simulink model "ADRCControl_20220610"  (R2020a)
settings: Solver=VariableStepAuto  StartTime=0.0  StopTime=12  FixedStep=0.01  RelTol=1e-3
values from neighbouring files (symbols this model uses):
  alpha1 = 0.5    [parameters_initialization.m]
  alpha2 = 0.25    [parameters_initialization.m]
  b = 2    [parameters_initialization.m]
  beta01 = 6    [parameters_initialization.m]
  beta02 = 24    [parameters_initialization.m]
  beta03 = 4    [parameters_initialization.m]
  delta = 0.0025    [parameters_initialization.m]
  h = 0.01    [parameters_initialization.m]
  h0 = 5 * h    (= 0.05)    [parameters_initialization.m]
  nlsef_alpha1 = 0.7    [parameters_initialization.m]
  nlsef_alpha2 = 1    [parameters_initialization.m]
  r = 100    [parameters_initialization.m]
undefined symbols (not defined in the file or in its folder): X, Y, Z
libraries: sm_lib x197, nesl_utility x84, sm_cable_robot_lib x44, simulink x3
(part 1 of 9)
settings Model: Creator=admin  LastModifiedBy=Administrator
settings SolverCC: AlgebraicLoopSolver=LineSearch

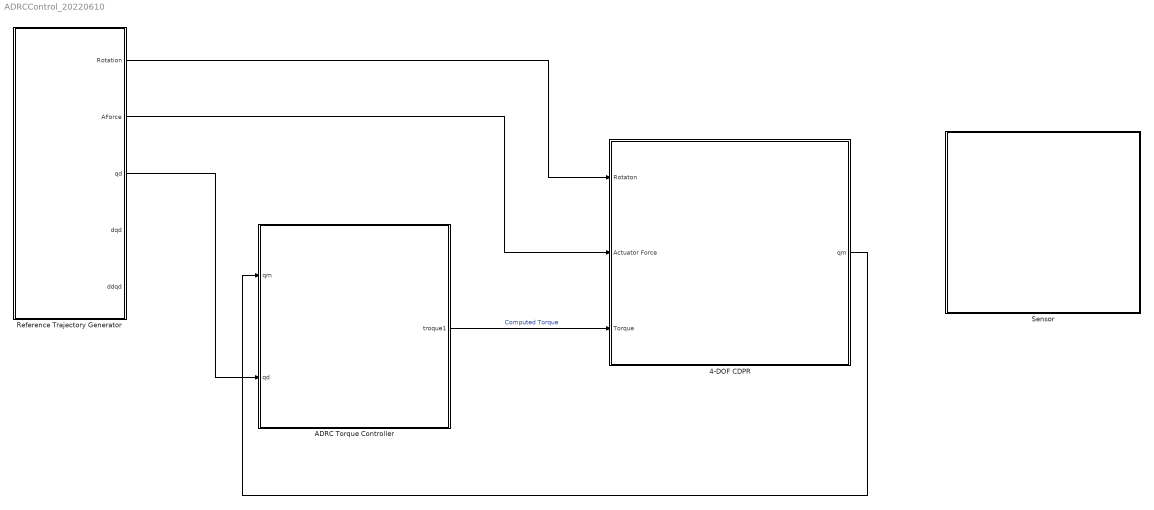
== system ADRCControl_20220610 ==
  4-DOF CDPR : Subsystem
  ADRC Torque Controller : Subsystem
  Reference Trajectory Generator : Subsystem
  Sensor : Subsystem
  wires:
  4-DOF CDPR/1(qm) -> ADRC Torque Controller/1(qm)
  Reference Trajectory Generator/1(Rotation) -> 4-DOF CDPR/1(Rotaton)
  Reference Trajectory Generator/2(AForce) -> 4-DOF CDPR/2("Actuator Force ")
  ADRC Torque Controller/1(troque1) -> 4-DOF CDPR/3(Torque)  "Computed Torque"
  Reference Trajectory Generator/3(qd) -> ADRC Torque Controller/2(qd)

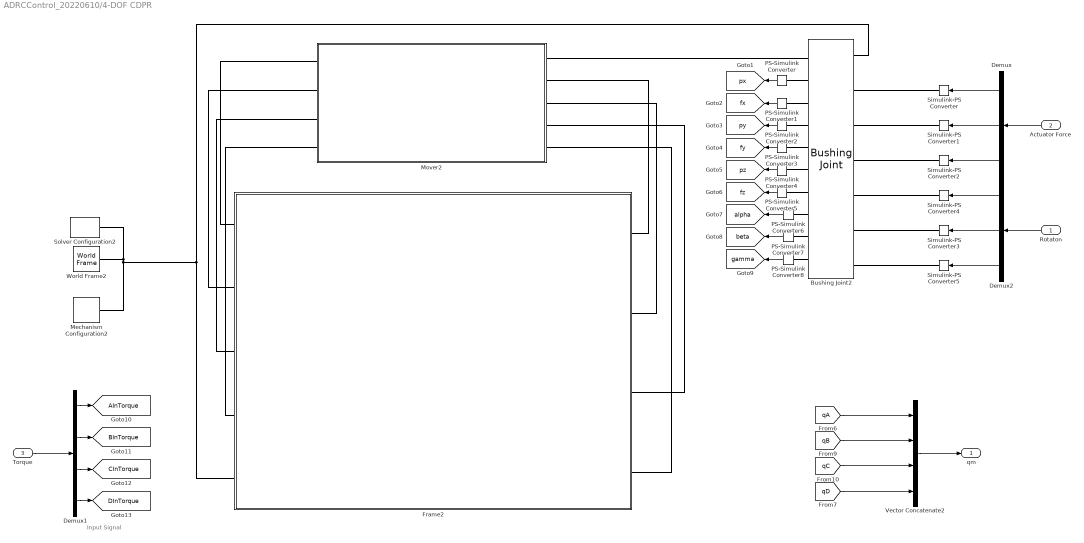
== system ADRCControl_20220610/4-DOF CDPR ==
  note: Input Signal
  Rotaton : Inport
  "Actuator Force " : Inport  Port=2
  Torque : Inport  Port=3
  Bushing Joint2 : sm_lib/Joints/Bushing Joint  JointMode=Normal  SenseConstraintForce=off  SenseConstraintForceX=off  SenseConstraintForceY=off  SenseConstraintForceZ=off  SenseConstraintTorque=off  SenseConstraintTorqueX=off  SenseConstraintTorqueY=off  SenseConstraintTorqueZ=off  SenseTotalForce=off  SenseTotalForceX=off  SenseTotalForceY=off  SenseTotalForceZ=off  SenseTotalTorque=off  SenseTotalTorqueX=off  SenseTotalTorqueY=off  SenseTotalTorqueZ=off  CompositeWrenchDir=FollowerOnBase  CompositeWrenchFrame=BaseFrame  PxEquilibriumPosition=0.2  PxEquilibriumPositionUnits=m  PxSpringStiffness=0  PxSpringStiffnessUnits=N/m  PxDampingCoefficient=0  PxDampingCoefficientUnits=N/(m/s)  PxTorqueActuationMode=InputTorque  PxMotionActuationMode=ComputedMotion  PxSensePosition=on  PxSenseVelocity=off  PxSenseAcceleration=off  PxSenseTorqueForce=on  PxSenseLowerLimitTorqueForce=off  PxSenseUpperLimitTorqueForce=off  PxLowerLimitSpecify=off  PxLowerLimitBound=-1  PxLowerLimitBoundUnits=m  PxLowerLimitStiffness=1e6  PxLowerLimitStiffnessUnits=N/m  PxLowerLimitDamping=1e3  PxLowerLimitDampingUnits=N/(m/s)  PxLowerLimitTransitionRegionWidth=1e-4  PxLowerLimitTransitionRegionWidthUnits=m  PxUpperLimitSpecify=off  PxUpperLimitBound=1  PxUpperLimitBoundUnits=m  PxUpperLimitStiffness=1e6  PxUpperLimitStiffnessUnits=N/m  PxUpperLimitDamping=1e3  PxUpperLimitDampingUnits=N/(m/s)  PxUpperLimitTransitionRegionWidth=1e-4  PxUpperLimitTransitionRegionWidthUnits=m  PxPositionTargetSpecify=on  PxPositionTargetPriority=Low  PxPositionTargetValue=0.2  PxPositionTargetValueUnits=m  PxVelocityTargetSpecify=off  PxVelocityTargetPriority=High  PxVelocityTargetValue=0.1047  PxVelocityTargetValueUnits=m/s  PyEquilibriumPosition=0  PyEquilibriumPositionUnits=m  PySpringStiffness=0  PySpringStiffnessUnits=N/m  PyDampingCoefficient=0  PyDampingCoefficientUnits=N/(m/s)  PyTorqueActuationMode=InputTorque  PyMotionActuationMode=ComputedMotion  PySensePosition=on  PySenseVelocity=off  PySenseAcceleration=off  PySenseTorqueForce=on  PySenseLowerLimitTorqueForce=off  PySenseUpperLimitTorqueForce=off  PyLowerLimitSpecify=off  PyLowerLimitBound=-1  PyLowerLimitBoundUnits=m  PyLowerLimitStiffness=1e6  PyLowerLimitStiffnessUnits=N/m  PyLowerLimitDamping=1e3  PyLowerLimitDampingUnits=N/(m/s)  PyLowerLimitTransitionRegionWidth=1e-4  PyLowerLimitTransitionRegionWidthUnits=m  PyUpperLimitSpecify=off  PyUpperLimitBound=1  PyUpperLimitBoundUnits=m  PyUpperLimitStiffness=1e6  PyUpperLimitStiffnessUnits=N/m  PyUpperLimitDamping=1e3  PyUpperLimitDampingUnits=N/(m/s)  PyUpperLimitTransitionRegionWidth=1e-4  PyUpperLimitTransitionRegionWidthUnits=m  PyPositionTargetSpecify=on  PyPositionTargetPriority=Low  PyPositionTargetValue=0  PyPositionTargetValueUnits=m  PyVelocityTargetSpecify=off  PyVelocityTargetPriority=High  PyVelocityTargetValue=0.1047  PyVelocityTargetValueUnits=m/s  PzEquilibriumPosition=1.3  PzEquilibriumPositionUnits=m  PzSpringStiffness=0  PzSpringStiffnessUnits=N/m  PzDampingCoefficient=0  PzDampingCoefficientUnits=N/(m/s)  PzTorqueActuationMode=InputTorque  PzMotionActuationMode=ComputedMotion  PzSensePosition=on  PzSenseVelocity=off  PzSenseAcceleration=off  PzSenseTorqueForce=on  PzSenseLowerLimitTorqueForce=off  PzSenseUpperLimitTorqueForce=off  PzLowerLimitSpecify=off  PzLowerLimitBound=-1  PzLowerLimitBoundUnits=m  PzLowerLimitStiffness=1e6  PzLowerLimitStiffnessUnits=N/m  PzLowerLimitDamping=1e3  PzLowerLimitDampingUnits=N/(m/s)  PzLowerLimitTransitionRegionWidth=1e-4  PzLowerLimitTransitionRegionWidthUnits=m  PzUpperLimitSpecify=off  PzUpperLimitBound=1  PzUpperLimitBoundUnits=m  PzUpperLimitStiffness=1e6  PzUpperLimitStiffnessUnits=N/m  PzUpperLimitDamping=1e3  PzUpperLimitDampingUnits=N/(m/s)  PzUpperLimitTransitionRegionWidth=1e-4  PzUpperLimitTransitionRegionWidthUnits=m  PzPositionTargetSpecify=on  PzPositionTargetPriority=Low  PzPositionTargetValue=1.3  PzPositionTargetValueUnits=m  PzVelocityTargetSpecify=off  PzVelocityTargetPriority=High  PzVelocityTargetValue=0  PzVelocityTargetValueUnits=m/s  RxEquilibriumPosition=0  RxEquilibriumPositionUnits=deg  RxSpringStiffness=0  RxSpringStiffnessUnits=N*m/deg  RxDampingCoefficient=0  RxDampingCoefficientUnits=N*m/(deg/s)  RxTorqueActuationMode=ComputedTorque  RxMotionActuationMode=InputMotion  RxSensePosition=on  RxSenseVelocity=off  RxSenseAcceleration=off  RxSenseTorqueForce=off  RxSenseLowerLimitTorqueForce=off  RxSenseUpperLimitTorqueForce=off  RxLowerLimitSpecify=off  RxLowerLimitBound=-90  RxLowerLimitBoundUnits=deg  RxLowerLimitStiffness=1e4  RxLowerLimitStiffnessUnits=N*m/deg  RxLowerLimitDamping=10  RxLowerLimitDampingUnits=N*m/(deg/s)  RxLowerLimitTransitionRegionWidth=0.1  RxLowerLimitTransitionRegionWidthUnits=deg  RxUpperLimitSpecify=off  RxUpperLimitBound=90  RxUpperLimitBoundUnits=deg  RxUpperLimitStiffness=1e4  RxUpperLimitStiffnessUnits=N*m/deg  RxUpperLimitDamping=10  RxUpperLimitDampingUnits=N*m/(deg/s)  RxUpperLimitTransitionRegionWidth=0.1  RxUpperLimitTransitionRegionWidthUnits=deg  RxPositionTargetSpecify=off  RxPositionTargetPriority=High  RxPositionTargetValue=0  RxPositionTargetValueUnits=deg  RxVelocityTargetSpecify=off  RxVelocityTargetPriority=High  RxVelocityTargetValue=0  RxVelocityTargetValueUnits=deg/s  RyEquilibriumPosition=0  RyEquilibriumPositionUnits=deg  RySpringStiffness=0  RySpringStiffnessUnits=N*m/deg  RyDampingCoefficient=0  RyDampingCoefficientUnits=N*m/(deg/s)  RyTorqueActuationMode=ComputedTorque  RyMotionActuationMode=InputMotion  RySensePosition=on  RySenseVelocity=off  RySenseAcceleration=off  RySenseTorqueForce=off  RySenseLowerLimitTorqueForce=off  RySenseUpperLimitTorqueForce=off  RyLowerLimitSpecify=off  RyLowerLimitBound=-90  RyLowerLimitBoundUnits=deg  RyLowerLimitStiffness=1e4  RyLowerLimitStiffnessUnits=N*m/deg  RyLowerLimitDamping=10  RyLowerLimitDampingUnits=N*m/(deg/s)  RyLowerLimitTransitionRegionWidth=0.1  RyLowerLimitTransitionRegionWidthUnits=deg  RyUpperLimitSpecify=off  RyUpperLimitBound=90  RyUpperLimitBoundUnits=deg  RyUpperLimitStiffness=1e4  RyUpperLimitStiffnessUnits=N*m/deg  RyUpperLimitDamping=10  RyUpperLimitDampingUnits=N*m/(deg/s)  RyUpperLimitTransitionRegionWidth=0.1  RyUpperLimitTransitionRegionWidthUnits=deg  RyPositionTargetSpecify=off  RyPositionTargetPriority=High  RyPositionTargetValue=0  RyPositionTargetValueUnits=deg  RyVelocityTargetSpecify=off  RyVelocityTargetPriority=High  RyVelocityTargetValue=0  RyVelocityTargetValueUnits=deg/s  RzEquilibriumPosition=0  RzEquilibriumPositionUnits=deg  RzSpringStiffness=0  RzSpringStiffnessUnits=N*m/deg  RzDampingCoefficient=0.01  RzDampingCoefficientUnits=N*m/(deg/s)  RzTorqueActuationMode=ComputedTorque  RzMotionActuationMode=InputMotion  RzSensePosition=on  RzSenseVelocity=off  RzSenseAcceleration=off  RzSenseTorqueForce=off  RzSenseLowerLimitTorqueForce=off  RzSenseUpperLimitTorqueForce=off  RzLowerLimitSpecify=off  RzLowerLimitBound=-90  RzLowerLimitBoundUnits=deg  RzLowerLimitStiffness=1e4  RzLowerLimitStiffnessUnits=N*m/deg  RzLowerLimitDamping=10  RzLowerLimitDampingUnits=N*m/(deg/s)  RzLowerLimitTransitionRegionWidth=0.1  RzLowerLimitTransitionRegionWidthUnits=deg  RzUpperLimitSpecify=off  RzUpperLimitBound=90  RzUpperLimitBoundUnits=deg  RzUpperLimitStiffness=1e4  RzUpperLimitStiffnessUnits=N*m/deg  RzUpperLimitDamping=10  RzUpperLimitDampingUnits=N*m/(deg/s)  RzUpperLimitTransitionRegionWidth=0.1  RzUpperLimitTransitionRegionWidthUnits=deg  RzPositionTargetSpecify=on  RzPositionTargetPriority=High  RzPositionTargetValue=0  RzPositionTargetValueUnits=deg  RzVelocityTargetSpecify=off  RzVelocityTargetPriority=High  RzVelocityTargetValue=0  RzVelocityTargetValueUnits=deg/s
  Demux : Demux  Outputs=3
  Demux1 : Demux
  Demux2 : Demux  Outputs=3
  Frame2 : Subsystem
  Mechanism Configuration2 : sm_lib/Utilities/Mechanism Configuration  UniformGravity=Constant  GravityVector=[0 0 -9.8]  GravityUnits=m/s^2  LinearizationDelta=0.001
  Mover2 : Subsystem
  PS-Simulink Converter{,1..8} (9 alike) : nesl_utility/PS-Simulink Converter  PhysicalDomain=network_engine_domain  SubClassName=ps_output  LeftPortType=input  RightPortType=output  PseudoPeriodic=off  Frequencies=[]  Unit=inherit  AffineConversion=off
  Simulink-PS Converter : nesl_utility/Simulink-PS Converter  PhysicalDomain=network_engine_domain  SubClassName=ps_input  LeftPortType=input  RightPortType=output  PseudoPeriodic=off  Frequencies=[]  NoiseDistribution=none  NoiseParameters=[]  Unit=N  AffineConversion=off  FilteringAndDerivatives=filter  SimscapeFilterOrder=2  InputFilterTimeConstant=0.001  UdotUserProvided=0
  Simulink-PS Converter1 : nesl_utility/Simulink-PS Converter  PhysicalDomain=network_engine_domain  SubClassName=ps_input  LeftPortType=input  RightPortType=output  PseudoPeriodic=off  Frequencies=[]  NoiseDistribution=none  NoiseParameters=[]  Unit=N  AffineConversion=off  FilteringAndDerivatives=filter  SimscapeFilterOrder=2  InputFilterTimeConstant=0.001  UdotUserProvided=0
  Simulink-PS Converter2 : nesl_utility/Simulink-PS Converter  PhysicalDomain=network_engine_domain  SubClassName=ps_input  LeftPortType=input  RightPortType=output  PseudoPeriodic=off  Frequencies=[]  NoiseDistribution=none  NoiseParameters=[]  Unit=N  AffineConversion=off  FilteringAndDerivatives=filter  SimscapeFilterOrder=2  InputFilterTimeConstant=0.001  UdotUserProvided=0
  Simulink-PS Converter3 : nesl_utility/Simulink-PS Converter  PhysicalDomain=network_engine_domain  SubClassName=ps_input  LeftPortType=input  RightPortType=output  PseudoPeriodic=off  Frequencies=[]  NoiseDistribution=none  NoiseParameters=[]  Unit=1  AffineConversion=off  FilteringAndDerivatives=filter  SimscapeFilterOrder=2  InputFilterTimeConstant=0.001  UdotUserProvided=0
  Simulink-PS Converter4 : nesl_utility/Simulink-PS Converter  PhysicalDomain=network_engine_domain  SubClassName=ps_input  LeftPortType=input  RightPortType=output  PseudoPeriodic=off  Frequencies=[]  NoiseDistribution=none  NoiseParameters=[]  Unit=1  AffineConversion=off  FilteringAndDerivatives=filter  SimscapeFilterOrder=2  InputFilterTimeConstant=0.001  UdotUserProvided=0
  Simulink-PS Converter5 : nesl_utility/Simulink-PS Converter  PhysicalDomain=network_engine_domain  SubClassName=ps_input  LeftPortType=input  RightPortType=output  PseudoPeriodic=off  Frequencies=[]  NoiseDistribution=none  NoiseParameters=[]  Unit=1  AffineConversion=off  FilteringAndDerivatives=filter  SimscapeFilterOrder=2  InputFilterTimeConstant=0.001  UdotUserProvided=0
  Solver Configuration2 : nesl_utility/Solver Configuration  PhysicalDomain=network_engine_domain  SubClassName=solver  LeftPortType=input  RightPortType=generic  Tones=[]  Harmonics=[]  SimulateNoise=off  Profile=off  UseLocalSampling=off  EnableSwitchedLinearOptims=on  FrequencyDomain=off  UseCCode=off  RelTol=0.001  AbsTol=1e-06  MinStep=1e-09  ToWorkspace=off  RevertToSquareIcSolve=off  NumHomotopyIterations=100  PhasorMode=off  PhasorModeNumHarmonics=1  DoDC=off  ResidualTolerance=1e-01  UseLocalSolver=off  LocalSolverChoice=NE_BACKWARD_EULER_ADVANCER  LocalSolverSampleTime=0.001  DoFixedCost=off  MaxNonlinIter=3  MaxModeIter=2  LinearAlgebra=Sparse  EquationFormulation=NE_TIME_EF  DelaysMemoryBudget=1024  AutomaticFiltering=on  FilteringTimeConstant=0.001  PartitionStorageMethod=AS_NEEDED  PartitionMemoryBudget=1024  PartitionMethod=ROBUST
  Vector Concatenate2 : Concatenate  NumInputs=4
  World Frame2 : sm_lib/Frames and Transforms/World Frame
  qm : Outport
  tag scope: AInTorque=global, BInTorque=global, CInTorque=global, DInTorque=global, alpha=global, beta=global, fx=global, fy=global, fz=global, gamma=global, px=global, py=global, pz=global
  wires:
  PS-Simulink Converter/1 -> [px]
  PS-Simulink Converter1/1 -> [fx]
  PS-Simulink Converter2/1 -> [py]
  PS-Simulink Converter4/1 -> [pz]
  PS-Simulink Converter3/1 -> [fy]
  PS-Simulink Converter5/1 -> [fz]
  PS-Simulink Converter7/1 -> [beta]
  PS-Simulink Converter6/1 -> [alpha]
  PS-Simulink Converter8/1 -> [gamma]
  Demux/2 -> Simulink-PS Converter1/1
  Demux/1 -> Simulink-PS Converter/1
  Demux/3 -> Simulink-PS Converter2/1
  "Actuator Force "/1 -> Demux/1
  Demux1/3 -> [CInTorque]
  Demux1/1 -> [AInTorque]
  Demux1/4 -> [DInTorque]
  Demux1/2 -> [BInTorque]
  Torque/1 -> Demux1/1
  Demux2/1 -> Simulink-PS Converter4/1
  Demux2/2 -> Simulink-PS Converter3/1
  Demux2/3 -> Simulink-PS Converter5/1
  Rotaton/1 -> Demux2/1
  Vector Concatenate2/1 -> qm/1
  [qC] -> Vector Concatenate2/3
  [qD] -> Vector Concatenate2/4
  [qA] -> Vector Concatenate2/1
  [qB] -> Vector Concatenate2/2
  connections:
  Frame2/RConn1 -- Mover2/RConn2
  Mover2/LConn3 -- Frame2/LConn3
  Mover2/LConn2 -- Frame2/LConn2
  Mover2/RConn4 -- Frame2/RConn3
  Frame2/LConn1 -- Mover2/LConn1
  Frame2/RConn2 -- Mover2/RConn3
  Frame2/LConn5 -- Bushing Joint2/LConn1 -- World Frame2/RConn1 -- Solver Configuration2/RConn1 -- Mechanism Configuration2/RConn1
  Bushing Joint2/RConn1 -- Mover2/RConn1
  Mover2/RConn5 -- Frame2/RConn4
  Mover2/LConn4 -- Frame2/LConn4
  Bushing Joint2/RConn2 -- PS-Simulink Converter/LConn1
  Bushing Joint2/RConn3 -- PS-Simulink Converter1/LConn1
  PS-Simulink Converter2/LConn1 -- Bushing Joint2/RConn4
  PS-Simulink Converter4/LConn1 -- Bushing Joint2/RConn6
  PS-Simulink Converter3/LConn1 -- Bushing Joint2/RConn5
  PS-Simulink Converter5/LConn1 -- Bushing Joint2/RConn7
  Bushing Joint2/RConn9 -- PS-Simulink Converter7/LConn1
  Bushing Joint2/RConn8 -- PS-Simulink Converter6/LConn1
  Bushing Joint2/RConn10 -- PS-Simulink Converter8/LConn1
  Simulink-PS Converter/RConn1 -- Bushing Joint2/LConn2
  Simulink-PS Converter1/RConn1 -- Bushing Joint2/LConn3
  Simulink-PS Converter2/RConn1 -- Bushing Joint2/LConn4
  Bushing Joint2/LConn5 -- Simulink-PS Converter4/RConn1
  Bushing Joint2/LConn6 -- Simulink-PS Converter3/RConn1
  Simulink-PS Converter5/RConn1 -- Bushing Joint2/LConn7

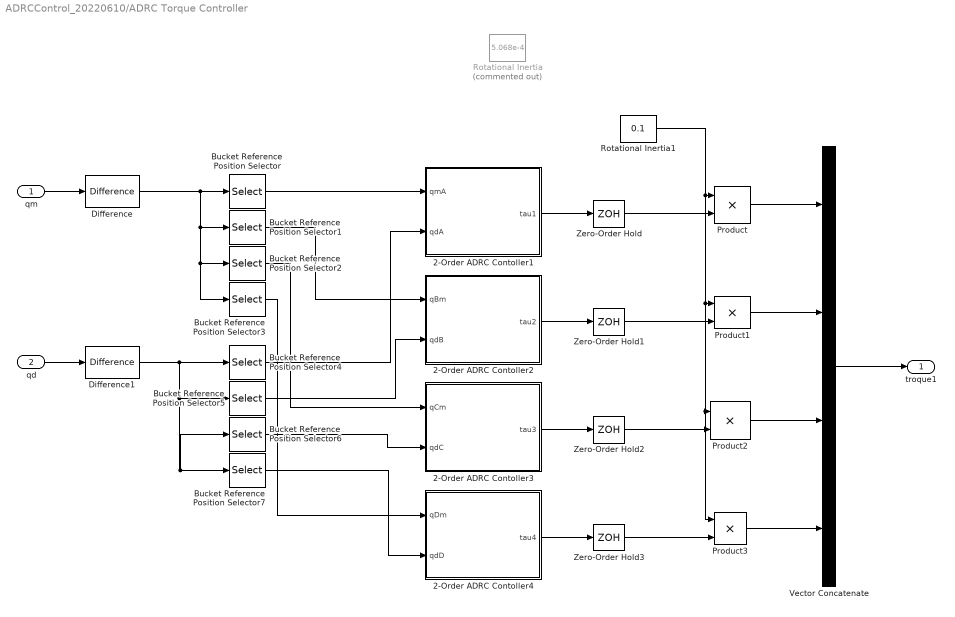
== system ADRCControl_20220610/ADRC Torque Controller ==
  qm : Inport
  qd : Inport  Port=2
  "2-Order ADRC Contoller1 " : Subsystem
  2-Order ADRC Contoller2 : Subsystem
  2-Order ADRC Contoller3 : Subsystem
  2-Order ADRC Contoller4 : Subsystem
  Bucket Reference Position Selector : Selector  InputPortWidth=4  IndexOptions=Index vector (dialog)  Indices=1  OutputSizes=1
  Bucket Reference Position Selector1 : Selector  InputPortWidth=4  IndexOptions=Index vector (dialog)  Indices=2  OutputSizes=1
  Bucket Reference Position Selector2 : Selector  InputPortWidth=4  IndexOptions=Index vector (dialog)  Indices=3  OutputSizes=1
  Bucket Reference Position Selector3 : Selector  InputPortWidth=4  IndexOptions=Index vector (dialog)  Indices=4  OutputSizes=1
  Bucket Reference Position Selector4 : Selector  InputPortWidth=4  IndexOptions=Index vector (dialog)  Indices=1  OutputSizes=1
  Bucket Reference Position Selector5 : Selector  InputPortWidth=4  IndexOptions=Index vector (dialog)  Indices=2  OutputSizes=1
  Bucket Reference Position Selector6 : Selector  InputPortWidth=4  IndexOptions=Index vector (dialog)  Indices=3  OutputSizes=1
  Bucket Reference Position Selector7 : Selector  InputPortWidth=4  IndexOptions=Index vector (dialog)  Indices=4  OutputSizes=1
  Difference : simulink/Discrete/Difference  ICPrevInput=0.0  OutMin=[]  OutMax=[]  OutDataType=fixdt(1, 16)  OutScaling=2^-10  DoSatur=off
  Difference1 : simulink/Discrete/Difference  ICPrevInput=0.0  OutMin=[]  OutMax=[]  OutDataType=fixdt(1, 16)  OutScaling=2^-10  DoSatur=off
  Product{,1..3} (4 alike) : Product
  Rotational Inertia : Constant  Commented=on  Value=5.068e-4
  Rotational Inertia1 : Constant  Value=0.1
  Vector Concatenate : Concatenate  NumInputs=4
  Zero-Order Hold{,1..3} (4 alike) : ZeroOrderHold  SampleTime=-1
  troque1 : Outport  VectorParamsAs1DForOutWhenUnconnected=off
  wires:
  qm/1 -> Difference/1
  Bucket Reference Position Selector/1 -> "2-Order ADRC Contoller1 "/1(qmA)
  Bucket Reference Position Selector1/1 -> 2-Order ADRC Contoller2/1(qBm)
  qd/1 -> Difference1/1
  Bucket Reference Position Selector2/1 -> 2-Order ADRC Contoller3/1(qCm)
  Bucket Reference Position Selector3/1 -> 2-Order ADRC Contoller4/1(qDm)
  Bucket Reference Position Selector4/1 -> "2-Order ADRC Contoller1 "/2(qdA)
  Bucket Reference Position Selector5/1 -> 2-Order ADRC Contoller2/2(qdB)
  Bucket Reference Position Selector6/1 -> 2-Order ADRC Contoller3/2(qdC)
  Bucket Reference Position Selector7/1 -> 2-Order ADRC Contoller4/2(qdD)
  Vector Concatenate/1 -> troque1/1
  Rotational Inertia1/1 -> Product3/1, Product2/1, Product1/1, Product/1
  Product/1 -> Vector Concatenate/1
  "2-Order ADRC Contoller1 "/1(tau1) -> Zero-Order Hold/1
  2-Order ADRC Contoller2/1(tau2) -> Zero-Order Hold1/1
  Product1/1 -> Vector Concatenate/2
  2-Order ADRC Contoller3/1(tau3) -> Zero-Order Hold2/1
  Product2/1 -> Vector Concatenate/3
  2-Order ADRC Contoller4/1(tau4) -> Zero-Order Hold3/1
  Product3/1 -> Vector Concatenate/4
  Zero-Order Hold/1 -> Product/2
  Zero-Order Hold1/1 -> Product1/2
  Zero-Order Hold2/1 -> Product2/2
  Zero-Order Hold3/1 -> Product3/2
  Difference/1 -> Bucket Reference Position Selector3/1, Bucket Reference Position Selector2/1, Bucket Reference Position Selector1/1, Bucket Reference Position Selector/1
  Difference1/1 -> Bucket Reference Position Selector7/1, Bucket Reference Position Selector6/1, Bucket Reference Position Selector5/1, Bucket Reference Position Selector4/1

== system ADRCControl_20220610/Reference Trajectory Generator ==
  Clock : Clock
      settings: Decimation=12
  Desired Angle : Subsystem
  End Actuator Force : Subsystem
  End Actuator Motion : Subsystem
  Rotation : Outport
  AForce : Outport  Port=2
  qd : Outport  Port=3
  dqd : Outport  Port=4
  ddqd : Outport  Port=5
  wires:
  Desired Angle/3(ddqd) -> ddqd/1
  Clock/1 -> Desired Angle/1(t)
  End Actuator Force/1(AForce) -> AForce/1
  Desired Angle/1(qd) -> qd/1
  End Actuator Motion/1(Rotation) -> Rotation/1
  Desired Angle/2(dqd) -> dqd/1

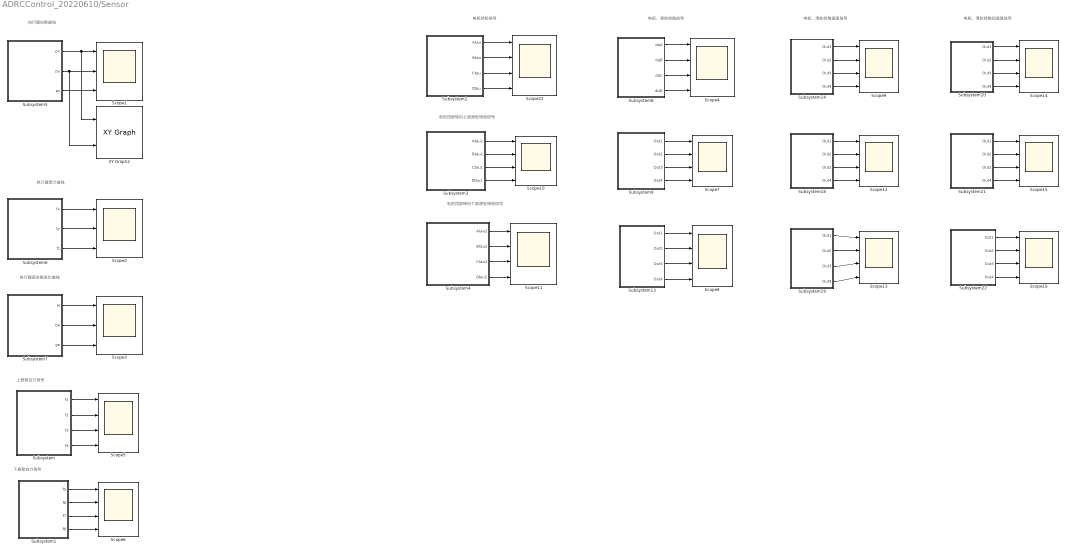
== system ADRCControl_20220610/Sensor ==
  note: 下悬索拉力信号
  note: 上悬索拉力信号
  note: 电机转矩信号
  note: 电机顶部转向上部滑轮转矩信号
  note: 电机顶部转向下部滑轮转矩信号
  note: 执行器位移曲线
  note: 执行器受力曲线
  note: 执行器姿态角变化曲线
  note: 电机、滑轮转角信号
  note: 电机、滑轮转角速度信号
  note: 电机、滑轮转角加速度信号
  Scope1 : Scope  NumInputPorts=3
  Scope{4..16,22} (14 alike) : Scope  NumInputPorts=4
  Scope2 : Scope  NumInputPorts=3
  Scope3 : Scope  NumInputPorts=3
  Subsystem : Subsystem
  Subsystem1 : Subsystem
  Subsystem13 : Subsystem
  Subsystem14 : Subsystem
  Subsystem18 : Subsystem
  Subsystem19 : Subsystem
  Subsystem2 : Subsystem
  Subsystem20 : Subsystem
  Subsystem21 : Subsystem
  Subsystem22 : Subsystem
  Subsystem3 : Subsystem
  Subsystem4 : Subsystem
  Subsystem5 : Subsystem
  Subsystem6 : Subsystem
  Subsystem7 : Subsystem
  Subsystem8 : Subsystem
  Subsystem9 : Subsystem
  XY Graph2 : simulink/Sinks/XY Graph  xmin=-1.1  xmax=1.1  ymin=-1.5  ymax=1.5  st=-1
  wires:
  Subsystem1/4(f8) -> Scope6/4
  Subsystem/1(f1) -> Scope5/1
  Subsystem1/3(f7) -> Scope6/3
  Subsystem/3(f3) -> Scope5/3
  Subsystem1/2(f6) -> Scope6/2
  Subsystem1/1(f5) -> Scope6/1
  Subsystem/2(f2) -> Scope5/2
  Subsystem/4(f4) -> Scope5/4
  Subsystem2/4(Dtau) -> Scope22/4
  Subsystem2/3(Ctau) -> Scope22/3
  Subsystem2/2(Btau) -> Scope22/2
  Subsystem2/1(Atau) -> Scope22/1
  Subsystem4/4(Dtau2) -> Scope11/4
  Subsystem4/3(Ctau2) -> Scope11/3
  Subsystem4/2(Btau2) -> Scope11/2
  Subsystem4/1(Atau2) -> Scope11/1
  Subsystem3/4(Dtau1) -> Scope10/4
  Subsystem3/1(Atau1) -> Scope10/1
  Subsystem3/3(Ctau1) -> Scope10/3
  Subsystem3/2(Btau1) -> Scope10/2
  Subsystem5/1(px) -> XY Graph2/1, Scope1/1
  Subsystem5/2(py) -> XY Graph2/2, Scope1/2
  Subsystem5/3(pz) -> Scope1/3
  Subsystem6/1(fx) -> Scope2/1
  Subsystem6/2(fy) -> Scope2/2
  Subsystem7/2(be) -> Scope3/2
  Subsystem6/3(fz) -> Scope2/3
  Subsystem7/1(al) -> Scope3/1
  Subsystem7/3(ga) -> Scope3/3
  Subsystem8/1(dqA) -> Scope4/1
  Subsystem8/2(dqB) -> Scope4/2
  Subsystem8/3(dqC) -> Scope4/3
  Subsystem8/4(dqD) -> Scope4/4
  Subsystem9/2(Out2) -> Scope7/2
  Subsystem9/1(Out1) -> Scope7/1
  Subsystem9/3(Out3) -> Scope7/3
  Subsystem9/4(Out4) -> Scope7/4
  Subsystem13/1(Out1) -> Scope8/1
  Subsystem13/2(Out2) -> Scope8/2
  Subsystem13/3(Out3) -> Scope8/3
  Subsystem13/4(Out4) -> Scope8/4
  Subsystem14/1(Out1) -> Scope9/1
  Subsystem14/2(Out2) -> Scope9/2
  Subsystem14/3(Out3) -> Scope9/3
  Subsystem14/4(Out4) -> Scope9/4
  Subsystem18/1(Out1) -> Scope12/1
  Subsystem18/2(Out2) -> Scope12/2
  Subsystem18/3(Out3) -> Scope12/3
  Subsystem18/4(Out4) -> Scope12/4
  Subsystem19/1(Out1) -> Scope13/1
  Subsystem19/2(Out2) -> Scope13/2
  Subsystem19/3(Out3) -> Scope13/3
  Subsystem19/4(Out4) -> Scope13/4
  Subsystem20/1(Out1) -> Scope14/1
  Subsystem20/2(Out2) -> Scope14/2
  Subsystem20/3(Out3) -> Scope14/3
  Subsystem20/4(Out4) -> Scope14/4
  Subsystem21/1(Out1) -> Scope15/1
  Subsystem21/2(Out2) -> Scope15/2
  Subsystem21/4(Out4) -> Scope15/4
  Subsystem21/3(Out3) -> Scope15/3
  Subsystem22/1(Out1) -> Scope16/1
  Subsystem22/2(Out2) -> Scope16/2
  Subsystem22/3(Out3) -> Scope16/3
  Subsystem22/4(Out4) -> Scope16/4

== system ADRCControl_20220610/4-DOF CDPR/Frame2 ==
  Base : sm_lib/Body Elements/Brick Solid  GraphicAmbientColor=[0.15 0.15 0.15 1.0]  BasedOnType=Density  BrickDimensions=[2.2 3 0.05]  BrickDimensionUnits=m  CenterOfMass=[0 0 0]  CenterOfMassUnits=m  GraphicDiffuseColor=[0.5 0.5 0.5]  Density=1000  DensityUnits=kg/m^3  DoExposeReferenceFrame=off  GraphicEmissiveColor=[0.0 0.0 0.0 1.0]  ExportEntireGeometry=off  SerializedFrames=<Frames><Frame><Id>Frame1</Id><Value><Name>Column1</Name><Origin><Source>GeometricFeature</Source><FeatureName>-x -y +z point</FeatureName></Origin><PrimaryAxis><DefinedDirection>+Y</DefinedDirection><Source>ReferenceFrame</Source><SourceDirection>+Y</SourceDirection><FeatureName></FeatureName></PrimaryAxis><SecondaryAxis><DefinedDirection>+Z</DefinedDirection><Source>ReferenceFrame</Source><SourceDirection>+Z</SourceDirection><FeatureName></FeatureName></SecondaryAxis></Value></Frame><Frame><Id>Frame2</Id><Value><Name>Column2</Name><Origin><Source>GeometricFeature</Source><FeatureName>+x -y +z point</FeatureName></Origin><PrimaryAxis><DefinedDirection>+Z</DefinedDirection><Source>ReferenceFrame</Source><SourceDirection>+Z</SourceDirection><FeatureName></FeatureName></PrimaryAxis><SecondaryAxis><DefinedDirection>+X</DefinedDirection><Source>ReferenceFrame</Source><SourceDirection>+X</SourceDirection><FeatureName></FeatureName></SecondaryAxis></Value></Frame><Frame><Id>Frame3</Id><Value><Name>Column3</Name><Origin><Source>GeometricFeature</Source><FeatureName>+x +y +z point</FeatureName></Origin><PrimaryAxis><DefinedDirection>+Z</DefinedDirection><Source>ReferenceFrame</Source><SourceDirection>+Z</SourceDirection><FeatureName></FeatureName></PrimaryAxis><SecondaryAxis><DefinedDirection>-X</DefinedDirection><Source>ReferenceFrame</Source><SourceDirection>+X</SourceDirection><FeatureName></FeatureName></SecondaryAxis></Value></Frame><Frame><Id>Frame4</Id><Value><Name>Column4</Name><Origin><Source>GeometricFeature</Source><FeatureName>-x +y +z point</FeatureName></Origin><PrimaryAxis><DefinedDirection>+Z</DefinedDirection><Source>ReferenceFrame</Source><SourceDirection>+Z</SourceDirection><FeatureName></FeatureName></PrimaryAxis><SecondaryAxis><DefinedDirection>-X</DefinedDirection><Source>ReferenceFrame</Source><SourceDirection>+X</SourceDirection><FeatureName></FeatureName></SecondaryAxis></Value></Frame><Frame><Id>Frame5</Id><Value><Name>mover</Name><Origin><Source>ReferenceFrame</Source><FeatureName></FeatureName></Origin><PrimaryAxis><DefinedDirection>+Z</DefinedDirection><Source>ReferenceFrame</Source><SourceDirection>+Z</SourceDirection><FeatureName></FeatureName></PrimaryAxis><SecondaryAxis><DefinedDirection>+X</DefinedDirection><Source>ReferenceFrame</Source><SourceDirection>+X</SourceDirection><FeatureName></FeatureName></SecondaryAxis></Value></Frame></Frames>  MarkerShape=Sphere  MarkerSize=10  GraphicType=FromGeometry  InertiaType=CalculateFromGeometry  Mass=1  MassUnits=kg  MomentsOfInertia=[1 1 1]  MomentsOfInertiaUnits=kg*m^2  GraphicOpacity=1.0  ProductsOfInertia=[0 0 0]  ProductsOfInertiaUnits=kg*m^2  GraphicShininess=75  GraphicSpecularColor=[0.5 0.5 0.5 1.0]  GraphicVisPropType=SimpleVisualProperties
  Column 1 : Subsystem
  Column 2 : Subsystem
  Column 3 : Subsystem
  Column 4 : Subsystem
  R1 : PMIOPort  Side=Left
  R2 : PMIOPort  Port=2  Side=Left
  R3 : PMIOPort  Port=3  Side=Left
  R4 : PMIOPort  Port=4  Side=Left
  B : PMIOPort  Port=5  Side=Left
  R5 : PMIOPort  Port=6  Side=Right
  R6 : PMIOPort  Port=7  Side=Right
  R7 : PMIOPort  Port=8  Side=Right
  R8 : PMIOPort  Port=9  Side=Right
  connections:
  Base/RConn2 -- Column 4/LConn1
  R5/RConn1 -- Column 3/LConn1
  R6/RConn1 -- Column 3/LConn2
  R4/RConn1 -- Column 2/RConn2
  R8/RConn1 -- Column 4/RConn2
  Base/LConn3 -- B/RConn1
  R7/RConn1 -- Column 4/RConn1
  Base/LConn1 -- Column 1/RConn1
  Base/LConn2 -- Column 3/RConn1
  R3/RConn1 -- Column 2/RConn1
  R2/RConn1 -- Column 1/LConn2
  Base/RConn1 -- Column 2/LConn1
  R1/RConn1 -- Column 1/LConn1

== system ADRCControl_20220610/4-DOF CDPR/Mover2 ==
  Mover : sm_lib/Body Elements/Brick Solid  GraphicAmbientColor=[0.15 0.15 0.15 1.0]  BasedOnType=Density  BrickDimensions=[0.2 0.05 0.1]  BrickDimensionUnits=m  CenterOfMass=[0.1 0.025 0.05]  CenterOfMassUnits=m  GraphicDiffuseColor=[1.0 0.2 0.2]  Density=5000  DensityUnits=kg/m^3  DoExposeReferenceFrame=off  GraphicEmissiveColor=[0.0 0.0 0.0 1.0]  ExportEntireGeometry=off  SerializedFrames=<Frames><Frame><Id>Frame1</Id><Value><Name>R1</Name><Origin><Source>GeometricFeature</Source><FeatureName>-x -y -z point</FeatureName></Origin><PrimaryAxis><DefinedDirection>+Z</DefinedDirection><Source>ReferenceFrame</Source><SourceDirection>+Z</SourceDirection><FeatureName></FeatureName></PrimaryAxis><SecondaryAxis><DefinedDirection>+X</DefinedDirection><Source>ReferenceFrame</Source><SourceDirection>+X</SourceDirection><FeatureName></FeatureName></SecondaryAxis></Value></Frame><Frame><Id>Frame2</Id><Value><Name>R5</Name><Origin><Source>GeometricFeature</Source><FeatureName>+x +y -z point</FeatureName></Origin><PrimaryAxis><DefinedDirection>+Z</DefinedDirection><Source>ReferenceFrame</Source><SourceDirection>+Z</SourceDirection><FeatureName></FeatureName></PrimaryAxis><SecondaryAxis><DefinedDirection>+X</DefinedDirection><Source>ReferenceFrame</Source><SourceDirection>+X</SourceDirection><FeatureName></FeatureName></SecondaryAxis></Value></Frame><Frame><Id>Frame3</Id><Value><Name>R2</Name><Origin><Source>GeometricFeature</Source><FeatureName>-x -y +z point</FeatureName></Origin><PrimaryAxis><DefinedDirection>+Z</DefinedDirection><Source>ReferenceFrame</Source><SourceDirection>+Z</SourceDirection><FeatureName></FeatureName></PrimaryAxis><SecondaryAxis><DefinedDirection>+X</DefinedDirection><Source>ReferenceFrame</Source><SourceDirection>+X</SourceDirection><FeatureName></FeatureName></SecondaryAxis></Value></Frame><Frame><Id>Frame4</Id><Value><Name>R6</Name><Origin><Source>GeometricFeature</Source><FeatureName>+x +y +z point</FeatureName></Origin><PrimaryAxis><DefinedDirection>+Z</DefinedDirection><Source>ReferenceFrame</Source><SourceDirection>+Z</SourceDirection><FeatureName></FeatureName></PrimaryAxis><SecondaryAxis><DefinedDirection>+X</DefinedDirection><Source>ReferenceFrame</Source><SourceDirection>+X</SourceDirection><FeatureName></FeatureName></SecondaryAxis></Value></Frame><Frame><Id>Frame5</Id><Value><Name>R3</Name><Origin><Source>GeometricFeature</Source><FeatureName>+x -y -z point</FeatureName></Origin><PrimaryAxis><DefinedDirection>+Z</DefinedDirection><Source>ReferenceFrame</Source><SourceDirection>+Z</SourceDirection><FeatureName></FeatureName></PrimaryAxis><SecondaryAxis><DefinedDirection>+X</DefinedDirection><Source>ReferenceFrame</Source><SourceDirection>+X</SourceDirection><FeatureName></FeatureName></SecondaryAxis></Value></Frame><Frame><Id>Frame6</Id><Value><Name>R7</Name><Origin><Source>GeometricFeature</Source><FeatureName>-x +y -z point</FeatureName></Origin><PrimaryAxis><DefinedDirection>+Z</DefinedDirection><Source>ReferenceFrame</Source><SourceDirection>+Z</SourceDirection><FeatureName></FeatureName></PrimaryAxis><SecondaryAxis><DefinedDirection>+X</DefinedDirection><Source>ReferenceFrame</Source><SourceDirection>+X</SourceDirection><FeatureName></FeatureName></SecondaryAxis></Value></Frame><Frame><Id>Frame7</Id><Value><Name>R4</Name><Origin><Source>GeometricFeature</Source><FeatureName>+x -y +z point</FeatureName></Origin><PrimaryAxis><DefinedDirection>+Z</DefinedDirection><Source>ReferenceFrame</Source><SourceDirection>+Z</SourceDirection><FeatureName></FeatureName></PrimaryAxis><SecondaryAxis><DefinedDirection>+X</DefinedDirection><Source>ReferenceFrame</Source><SourceDirection>+X</SourceDirection><FeatureName></FeatureName></SecondaryAxis></Value></Frame><Frame><Id>Frame8</Id><Value><Name>R8</Name><Origin><Source>GeometricFeature</Source><FeatureName>-x +y +z point</FeatureName></Origin><PrimaryAxis><DefinedDirection>+Z</DefinedDirection><Source>ReferenceFrame</Source><SourceDirection>+Z</SourceDirection><FeatureName></FeatureName></PrimaryAxis><SecondaryAxis><DefinedDirection>+X</DefinedDirection><Source>ReferenceFrame</Source><SourceDirection>+X</SourceDirection><FeatureName></FeatureName></SecondaryAxis></Value></Frame><Frame><Id>Frame9</Id><Value><Name>R</Name><Origin><Source>ReferenceFrame</Source><FeatureName></FeatureName></Origin><PrimaryAxis><DefinedDirection>+Z</DefinedDirection><Source>ReferenceFrame</Source><SourceDirection>+Z</SourceDirection><FeatureName></FeatureName></PrimaryAxis><SecondaryAxis><DefinedDirection>+X</DefinedDirection><Source>ReferenceFrame</Source><SourceDirection>+X</SourceDirection><FeatureName></FeatureName></SecondaryAxis></Value></Frame></Frames>  MarkerShape=Sphere  MarkerSize=10  GraphicType=FromGeometry  InertiaType=Custom  Mass=5  MassUnits=kg  MomentsOfInertia=[1 1 1]  MomentsOfInertiaUnits=kg*m^2  GraphicOpacity=1.0  ProductsOfInertia=[0 0 0]  ProductsOfInertiaUnits=kg*m^2  GraphicShininess=75  GraphicSpecularColor=[0.5 0.5 0.5 1.0]  GraphicVisPropType=SimpleVisualProperties
  R1 : PMIOPort  Side=Left
  R2 : PMIOPort  Port=2  Side=Left
  R3 : PMIOPort  Port=3  Side=Left
  R4 : PMIOPort  Port=4  Side=Left
  R : PMIOPort  Port=5  Side=Right
  R5 : PMIOPort  Port=6  Side=Right
  R6 : PMIOPort  Port=7  Side=Right
  R7 : PMIOPort  Port=8  Side=Right
  R8 : PMIOPort  Port=9  Side=Right
  connections:
  R1/RConn1 -- Mover/LConn1
  R8/RConn1 -- Mover/RConn4
  R/RConn1 -- Mover/LConn5
  R7/RConn1 -- Mover/RConn3
  R4/RConn1 -- Mover/LConn4
  R6/RConn1 -- Mover/RConn2
  R2/RConn1 -- Mover/LConn2
  R5/RConn1 -- Mover/RConn1
  R3/RConn1 -- Mover/LConn3

== system ADRCControl_20220610/ADRC Torque Controller/2-Order ADRC Contoller1  ==
  qmA : Inport
  qdA : Inport  Port=2
  Divide : Product  Inputs=*/
  ESO : Subsystem
  NLSEF : Subsystem
  Sum : Sum  Inputs=|+-
  Sum1 : Sum  Inputs=|+-
  Sum2 : Sum  Inputs=|+-
  TD : Subsystem
  b : Constant  Value=b
  b1 : Gain  Gain=b
  tau1 : Outport  VectorParamsAs1DForOutWhenUnconnected=off
  wires:
  Sum1/1 -> NLSEF/2(e2)  "e2"
  TD/1(v1) -> Sum/1
  ESO/1(z3) -> Divide/1  "z3"
  NLSEF/1(u0) -> Sum2/1  "u0"
  TD/2(v2) -> Sum1/1
  Divide/1 -> Sum2/2
  Sum2/1 -> tau1/1, b1/1  "u"
  b/1 -> Divide/2
  b1/1 -> ESO/1(bu)
  Sum/1 -> NLSEF/1(e1)  "e1"
  ESO/3(z1) -> Sum/2  "z1"
  ESO/2(z2) -> Sum1/2  "z2"
  qmA/1 -> ESO/2(y)
  qdA/1 -> TD/1(v0)

== system ADRCControl_20220610/ADRC Torque Controller/2-Order ADRC Contoller2 ==
  qBm : Inport
  qdB : Inport  Port=2
  Divide : Product  Inputs=*/
  ESO : Subsystem
  NLSEF : Subsystem
  Sum : Sum  Inputs=|+-
  Sum1 : Sum  Inputs=|+-
  Sum2 : Sum  Inputs=|+-
  TD : Subsystem
  b : Constant  Value=b
  b1 : Gain  Gain=b
  tau2 : Outport  VectorParamsAs1DForOutWhenUnconnected=off
  wires:
  Sum1/1 -> NLSEF/2(e2)  "e2"
  TD/1(v1) -> Sum/1
  ESO/1(z3) -> Divide/1  "z3"
  NLSEF/1(u0) -> Sum2/1  "u0"
  TD/2(v2) -> Sum1/1
  Divide/1 -> Sum2/2
  Sum2/1 -> tau2/1, b1/1  "u"
  b/1 -> Divide/2
  b1/1 -> ESO/1(bu)
  Sum/1 -> NLSEF/1(e1)  "e1"
  ESO/3(z1) -> Sum/2  "z1"
  ESO/2(z2) -> Sum1/2  "z2"
  qBm/1 -> ESO/2(y)
  qdB/1 -> TD/1(v0)

== system ADRCControl_20220610/ADRC Torque Controller/2-Order ADRC Contoller3 ==
  qCm : Inport
  qdC : Inport  Port=2
  Divide : Product  Inputs=*/
  ESO : Subsystem
  NLSEF : Subsystem
  Sum : Sum  Inputs=|+-
  Sum1 : Sum  Inputs=|+-
  Sum2 : Sum  Inputs=|+-
  TD : Subsystem
  b : Constant  Value=b
  b1 : Gain  Gain=b
  tau3 : Outport  VectorParamsAs1DForOutWhenUnconnected=off
  wires:
  Sum1/1 -> NLSEF/2(e2)  "e2"
  TD/1(v1) -> Sum/1
  ESO/1(z3) -> Divide/1  "z3"
  NLSEF/1(u0) -> Sum2/1  "u0"
  TD/2(v2) -> Sum1/1
  Divide/1 -> Sum2/2
  Sum2/1 -> tau3/1, b1/1  "u"
  b/1 -> Divide/2
  b1/1 -> ESO/1(bu)
  Sum/1 -> NLSEF/1(e1)  "e1"
  ESO/3(z1) -> Sum/2  "z1"
  ESO/2(z2) -> Sum1/2  "z2"
  qCm/1 -> ESO/2(y)
  qdC/1 -> TD/1(v0)

== system ADRCControl_20220610/ADRC Torque Controller/2-Order ADRC Contoller4 ==
  qDm : Inport
  qdD : Inport  Port=2
  Divide : Product  Inputs=*/
  ESO : Subsystem
  NLSEF : Subsystem
  Sum : Sum  Inputs=|+-
  Sum1 : Sum  Inputs=|+-
  Sum2 : Sum  Inputs=|+-
  TD : Subsystem
  b : Constant  Value=b
  b1 : Gain  Gain=b
  tau4 : Outport  VectorParamsAs1DForOutWhenUnconnected=off
  wires:
  Sum1/1 -> NLSEF/2(e2)  "e2"
  TD/1(v1) -> Sum/1
  ESO/1(z3) -> Divide/1  "z3"
  NLSEF/1(u0) -> Sum2/1  "u0"
  TD/2(v2) -> Sum1/1
  Divide/1 -> Sum2/2
  Sum2/1 -> tau4/1, b1/1  "u"
  b/1 -> Divide/2
  b1/1 -> ESO/1(bu)
  Sum/1 -> NLSEF/1(e1)  "e1"
  ESO/3(z1) -> Sum/2  "z1"
  ESO/2(z2) -> Sum1/2  "z2"
  qDm/1 -> ESO/2(y)
  qdD/1 -> TD/1(v0)

== system ADRCControl_20220610/Reference Trajectory Generator/Desired Angle ==
  t : Inport
  MATLAB Function2 : MATLAB Function  TreatAsAtomicUnit=on
  MATLAB Function3 : MATLAB Function  TreatAsAtomicUnit=on
  MATLAB Function4 : MATLAB Function  TreatAsAtomicUnit=on
  Vector Concatenate : Concatenate  NumInputs=4
  Vector Concatenate1 : Concatenate  NumInputs=4
  Vector Concatenate2 : Concatenate  NumInputs=4
  qd : Outport
  dqd : Outport  Port=2
  ddqd : Outport  Port=3
  wires:
  Vector Concatenate2/1 -> ddqd/1
  Vector Concatenate/1 -> qd/1
  MATLAB Function4/2(Bq) -> Vector Concatenate/2
  MATLAB Function2/4(Ddq) -> Vector Concatenate1/4
  MATLAB Function4/1(Aq) -> Vector Concatenate/1
  MATLAB Function4/4(Dq) -> Vector Concatenate/4
  MATLAB Function2/1(Adq) -> Vector Concatenate1/1
  MATLAB Function4/3(Cq) -> Vector Concatenate/3
  MATLAB Function2/3(Cdq) -> Vector Concatenate1/3
  MATLAB Function3/1(Addq) -> Vector Concatenate2/1
  Vector Concatenate1/1 -> dqd/1
  MATLAB Function2/2(Bdq) -> Vector Concatenate1/2
  MATLAB Function3/3(Cddq) -> Vector Concatenate2/3
  MATLAB Function3/2(Bddq) -> Vector Concatenate2/2
  t/1 -> MATLAB Function4/1(t), MATLAB Function3/1(t), MATLAB Function2/1(t)

== system ADRCControl_20220610/Reference Trajectory Generator/End Actuator Force ==
  Px Signal : FromWorkspace  VariableName=mover.forceSignal.fx  ZeroCross=off  OutputAfterFinalValue=Holding final value
  Py Signal : FromWorkspace  VariableName=mover.forceSignal.fy  ZeroCross=off  OutputAfterFinalValue=Holding final value
  Pz Signal : FromWorkspace  VariableName=mover.forceSignal.fz  ZeroCross=off  OutputAfterFinalValue=Holding final value
  Vector Concatenate : Concatenate  NumInputs=3
  AForce : Outport  VectorParamsAs1DForOutWhenUnconnected=off
  wires:
  Py Signal/1 -> Vector Concatenate/2
  Px Signal/1 -> Vector Concatenate/1
  Pz Signal/1 -> Vector Concatenate/3
  Vector Concatenate/1 -> AForce/1

== system ADRCControl_20220610/Reference Trajectory Generator/End Actuator Motion ==
  Constant : Constant  Value=0
  Constant1 : Constant  Value=0
  Constant2 : Constant  Value=0
  Mux : Mux  Inputs=3
  Sum : Sum  Inputs=|-+
  Rotation : Outport
  wires:
  Constant/1 -> Mux/2
  Constant1/1 -> Mux/1
  [gamma] -> Sum/1
  Sum/1 -> Mux/3
  Constant2/1 -> Sum/2
  Mux/1 -> Rotation/1

== system ADRCControl_20220610/Sensor/Subsystem ==
  f1 : Outport
  f2 : Outport  Port=2
  f3 : Outport  Port=3
  f4 : Outport  Port=4
  wires:
  [f1] -> f1/1
  [f3] -> f3/1
  [f4] -> f4/1
  [f2] -> f2/1

== system ADRCControl_20220610/Sensor/Subsystem1 ==
  f5 : Outport
  f6 : Outport  Port=2
  f7 : Outport  Port=3
  f8 : Outport  Port=4
  wires:
  [f6] -> f6/1
  [f5] -> f5/1
  [f8] -> f8/1
  [f7] -> f7/1

== system ADRCControl_20220610/Sensor/Subsystem13 ==
  Out1 : Outport
  Out2 : Outport  Port=2
  Out3 : Outport  Port=3
  Out4 : Outport  Port=4
  wires:
  [dqD2] -> Out4/1
  [dqC2] -> Out3/1
  [dqA2] -> Out1/1
  [dqB2] -> Out2/1

== system ADRCControl_20220610/Sensor/Subsystem14 ==
  Out1 : Outport
  Out2 : Outport  Port=2
  Out3 : Outport  Port=3
  Out4 : Outport  Port=4
  wires:
  [qD] -> Out4/1
  [qB] -> Out2/1
  [qC] -> Out3/1
  [qA] -> Out1/1

== system ADRCControl_20220610/Sensor/Subsystem18 ==
  Out1 : Outport
  Out2 : Outport  Port=2
  Out3 : Outport  Port=3
  Out4 : Outport  Port=4
  wires:
  [qA1] -> Out1/1
  [qC1] -> Out3/1
  [qB1] -> Out2/1
  [qD1] -> Out4/1

== system ADRCControl_20220610/Sensor/Subsystem19 ==
  Out1 : Outport
  Out2 : Outport  Port=2
  Out3 : Outport  Port=3
  Out4 : Outport  Port=4
  wires:
  [qB2] -> Out2/1
  [qC2] -> Out3/1
  [qD2] -> Out4/1
  [qA2] -> Out1/1

== system ADRCControl_20220610/Sensor/Subsystem2 ==
  Atau : Outport
  Btau : Outport  Port=2
  Ctau : Outport  Port=3
  Dtau : Outport  Port=4
  wires:
  [Btrq] -> Btau/1
  [Ctrq] -> Ctau/1
  [Atrq] -> Atau/1
  [Dtrq] -> Dtau/1

== system ADRCControl_20220610/Sensor/Subsystem20 ==
  Out1 : Outport
  Out2 : Outport  Port=2
  Out3 : Outport  Port=3
  Out4 : Outport  Port=4
  wires:
  [ddqA] -> Out1/1
  [ddqB] -> Out2/1
  [ddqD] -> Out4/1
  [ddqC] -> Out3/1

== system ADRCControl_20220610/Sensor/Subsystem21 ==
  Out1 : Outport
  Out2 : Outport  Port=2
  Out3 : Outport  Port=3
  Out4 : Outport  Port=4
  wires:
  [ddqA1] -> Out1/1
  [ddqB1] -> Out2/1
  [ddqD1] -> Out4/1
  [ddqC1] -> Out3/1

== system ADRCControl_20220610/Sensor/Subsystem22 ==
  Out1 : Outport
  Out2 : Outport  Port=2
  Out3 : Outport  Port=3
  Out4 : Outport  Port=4
  wires:
  [ddqA2] -> Out1/1
  [ddqD2] -> Out4/1
  [ddqB2] -> Out2/1
  [ddqC2] -> Out3/1

== system ADRCControl_20220610/Sensor/Subsystem3 ==
  Atau1 : Outport
  Btau1 : Outport  Port=2
  Ctau1 : Outport  Port=3
  Dtau1 : Outport  Port=4
  wires:
  [Btrq1] -> Btau1/1
  [Ctrq1] -> Ctau1/1
  [Atrq1] -> Atau1/1
  [Dtrq1] -> Dtau1/1

== system ADRCControl_20220610/Sensor/Subsystem4 ==
  Atau2 : Outport
  Btau2 : Outport  Port=2
  Ctau2 : Outport  Port=3
  Dtau2 : Outport  Port=4
  wires:
  [Dtrq2] -> Dtau2/1
  [Atrq2] -> Atau2/1
  [Btrq2] -> Btau2/1
  [Ctrq2] -> Ctau2/1

== system ADRCControl_20220610/Sensor/Subsystem5 ==
  px : Outport
  py : Outport  Port=2
  pz : Outport  Port=3
  wires:
  [py] -> py/1
  [px] -> px/1
  [pz] -> pz/1

== system ADRCControl_20220610/Sensor/Subsystem6 ==
  fx : Outport
  fy : Outport  Port=2
  fz : Outport  Port=3
  wires:
  [fy] -> fy/1
  [fx] -> fx/1
  [fz] -> fz/1

== system ADRCControl_20220610/Sensor/Subsystem7 ==
  al : Outport
  be : Outport  Port=2
  ga : Outport  Port=3
  wires:
  [beta] -> be/1
  [alpha] -> al/1
  [gamma] -> ga/1

== system ADRCControl_20220610/Sensor/Subsystem8 ==
  dqA : Outport
  dqB : Outport  Port=2
  dqC : Outport  Port=3
  dqD : Outport  Port=4
  wires:
  [dqB] -> dqB/1
  [dqA] -> dqA/1
  [dqD] -> dqD/1
  [dqC] -> dqC/1

== system ADRCControl_20220610/Sensor/Subsystem9 ==
  Out1 : Outport
  Out2 : Outport  Port=2
  Out3 : Outport  Port=3
  Out4 : Outport  Port=4
  wires:
  [dqD1] -> Out4/1
  [dqA1] -> Out1/1
  [dqB1] -> Out2/1
  [dqC1] -> Out3/1
